simulink library "vehicle_model"  (R2018b)
settings: Solver=ode45  StartTime=0.0  StopTime=10.0  RelTol=1e-3  EnableMultiTasking=on
undefined symbols (not defined in the file): DiscIntNeverNeededParam, par_VEH, select_To_Wks_akt, stepsize, v0
libraries: $bdroot x8, pacejka_trans x6, simulink x4, body_chassis_vert x1
(part 4 of 4)

== system vehicle_model/vehicle_model/wheel/wheel_lift/wheel_lift_RR ==
  Fz_tire_wheel : Inport
  Fzt : Inport  Port=2
  z_init : Inport  Port=3
  Add : Sum  Inputs=+-
  Bus Creator : BusCreator  Inputs=3
  Discrete-Time Integrator : DiscreteIntegrator  ExternalReset=level  SampleTime=-1  ICPrevOutput=DiscIntNeverNeededParam  ICPrevScaledInput=DiscIntNeverNeededParam
  Discrete-Time Integrator1 : DiscreteIntegrator  ExternalReset=level  InitialConditionSource=external  SampleTime=-1  ICPrevOutput=DiscIntNeverNeededParam  ICPrevScaledInput=DiscIntNeverNeededParam
  Divide : Product  Inputs=*/
  Gain : Gain  Gain=0.5
  zwheel : Outport
  wires:
  Add/1 -> Divide/1
  Fz_tire_wheel/1 -> Add/1
  Fzt/1 -> Add/2
  Divide/1 -> Discrete-Time Integrator/1, Bus Creator/3  "zwheelpp"
  Discrete-Time Integrator/1 -> Discrete-Time Integrator1/1, Bus Creator/2  "zwheelp"
  Discrete-Time Integrator1/1 -> Bus Creator/1  "zwheel"
  Bus Creator/1 -> zwheel/1
  [m_usR] -> Gain/1
  Gain/1 -> Divide/2
  [reset] -> Discrete-Time Integrator/2, Discrete-Time Integrator1/2
  z_init/1 -> Discrete-Time Integrator1/3

== system vehicle_model/simplified_vehicle_model/body_chassis_vert/suspension/damper/Front ==
  z_pitchp : Inport
  z_vertp : Inport  Port=2
  z_wheel_vertp : Inport  Port=3
  Add : Sum  Inputs=++-
  Divide : Product  Inputs=*/
  Product1 : Product  RndMeth=Zero
  Product2 : Product  RndMeth=Zero
  Product3 : Product  RndMeth=Zero
  Switch : Switch
  compression : Polyval  Coefs=par_VEH.ddF_comp
  rebound : Polyval  Coefs=par_VEH.ddF_reb
  Fz_damper : Outport
  P_damper : Outport  Port=2
  wires:
  Product1/1 -> P_damper/1
  z_wheel_vertp/1 -> Add/3
  z_pitchp/1 -> Add/1
  z_vertp/1 -> Add/2
  [sdF] -> Divide/1
  [sF] -> Divide/2
  Divide/1 -> Product2/2, Product3/2
  Product2/1 -> Fz_damper/1
  compression/1 -> Switch/3
  rebound/1 -> Switch/1
  Switch/1 -> Product2/1, Product1/1
  Add/1 -> Product3/1
  Product3/1 -> Product1/2, compression/1, Switch/2, rebound/1

== system vehicle_model/simplified_vehicle_model/body_chassis_vert/suspension/damper/Rear ==
  z_pitchp : Inport
  z_vertp : Inport  Port=2
  z_wheel_vertp : Inport  Port=3
  Add : Sum  Inputs=++-
  Divide : Product  Inputs=*/
  Product1 : Product  RndMeth=Zero
  Product2 : Product  RndMeth=Zero
  Product3 : Product  RndMeth=Zero
  Switch : Switch
  compression : Polyval  Coefs=par_VEH.ddR_comp
  rebound : Polyval  Coefs=par_VEH.ddR_reb
  Fz_damper : Outport
  P_damper : Outport  Port=2
  wires:
  Product1/1 -> P_damper/1
  Product3/1 -> compression/1, Product1/2, rebound/1, Switch/2
  Switch/1 -> Product2/1, Product1/1
  z_wheel_vertp/1 -> Add/3
  z_pitchp/1 -> Add/1
  z_vertp/1 -> Add/2
  [sdR] -> Divide/1
  [sR] -> Divide/2
  Divide/1 -> Product3/2, Product2/2
  Product2/1 -> Fz_damper/1
  compression/1 -> Switch/3
  rebound/1 -> Switch/1
  Add/1 -> Product3/1

== system vehicle_model/simplified_vehicle_model/body_chassis_vert/suspension/spring/Front ==
  z_pitch : Inport
  z_vert : Inport  Port=2
  z_wheel_vert : Inport  Port=3
  Add : Sum  Inputs=--+
  Divide : Product  Inputs=*/
  Product : Product
  Product1 : Product
  csRF : Lookup_n-D  NumberOfTableDimensions=1  BreakpointsForDimension1=par_VEH.cF_front(:,1)  Table=par_VEH.cF_front(:,2)  InternalRulePriority=Speed  RndMeth=Simplest  InputSameDT=on
  Fz_spring : Outport
  z_wheel : Outport  Port=2
  wires:
  Product1/1 -> Fz_spring/1
  Add/1 -> Product/1, z_wheel/1
  z_pitch/1 -> Add/1
  z_vert/1 -> Add/2
  z_wheel_vert/1 -> Add/3
  [ssF] -> Divide/1
  [sF] -> Divide/2
  Product/1 -> csRF/1
  Divide/1 -> Product1/2, Product/2
  csRF/1 -> Product1/1

== system vehicle_model/simplified_vehicle_model/body_chassis_vert/suspension/spring/Rear ==
  z_pitch : Inport
  z_vert : Inport  Port=2
  z_wheel_vert : Inport  Port=3
  Add : Sum  Inputs=--+
  Divide : Product  Inputs=*/
  Product : Product
  Product1 : Product
  csRF : Lookup_n-D  NumberOfTableDimensions=1  BreakpointsForDimension1=par_VEH.cF_rear(:,1)  Table=par_VEH.cF_rear(:,2)  InternalRulePriority=Speed  RndMeth=Simplest  InputSameDT=on
  Fz_spring : Outport
  z_wheel : Outport  Port=2
  wires:
  csRF/1 -> Product1/1
  Add/1 -> Product/1, z_wheel/1
  z_pitch/1 -> Add/1
  z_vert/1 -> Add/2
  z_wheel_vert/1 -> Add/3
  [ssR] -> Divide/1
  [sR] -> Divide/2
  Divide/1 -> Product1/2, Product/2
  Product/1 -> csRF/1
  Product1/1 -> Fz_spring/1

== system vehicle_model/simplified_vehicle_model/wheel/calc_omega/friction/Begrenzung bei durchgehendem Rad ==
  omega : Inport
  Abs : Abs
  Bias : Bias  Bias=-350
  Bias1 : Bias  Bias=0.5
  Demux : Demux  Outputs=2
  Gain : Gain  Gain=1000
  Gain1 : Gain  Gain=0.5
  Gain2 : Gain  Gain=1/30
  Product : Product  RndMeth=Zero
  Sign : Signum
  Trigonometric Function : Trigonometry  Operator=tanh
  friction_F : Outport
  friction_R : Outport  Port=2
  wires:
  Gain/1 -> Product/1
  Demux/2 -> friction_R/1
  Demux/1 -> friction_F/1
  Product/1 -> Demux/1
  Sign/1 -> Product/2
  Bias1/1 -> Gain/1
  Gain2/1 -> Trigonometric Function/1
  Bias/1 -> Gain2/1
  Abs/1 -> Bias/1
  omega/1 -> Sign/1, Abs/1
  Trigonometric Function/1 -> Gain1/1
  Gain1/1 -> Bias1/1

== system vehicle_model/vehicle_model/wheel/calc_omega/friction/Begrenzung bei durchgehendem Rad ==
  omega : Inport
  Abs : Abs
  Bias : Bias  Bias=-350
  Bias1 : Bias  Bias=0.5
  Demux : Demux
  Gain : Gain  Gain=1000
  Gain1 : Gain  Gain=0.5
  Gain2 : Gain  Gain=1/30
  Product : Product  RndMeth=Zero
  Sign : Signum
  Trigonometric Function : Trigonometry  Operator=tanh
  friction_RF : Outport
  friction_LF : Outport  Port=2
  friction_RR : Outport  Port=3
  friction_LR : Outport  Port=4
  wires:
  Gain1/1 -> Bias1/1
  Trigonometric Function/1 -> Gain1/1
  omega/1 -> Abs/1, Sign/1
  Abs/1 -> Bias/1
  Bias/1 -> Gain2/1
  Gain2/1 -> Trigonometric Function/1
  Bias1/1 -> Gain/1
  Sign/1 -> Product/2
  Product/1 -> Demux/1
  Demux/1 -> friction_RF/1
  Demux/2 -> friction_LF/1
  Demux/3 -> friction_RR/1
  Demux/4 -> friction_LR/1
  Gain/1 -> Product/1
